simulink model "SMC"  (R2013b)
settings: Solver=ode45  StartTime=0.0  StopTime=50  RelTol=1e-3
InitFcn:
  | params
StartFcn:
  | params
undefined symbols (not defined in the file or in its folder): P, SM_controller
settings Model: Creator=dave  LastModifiedBy=dave
settings DataIOCC: SignalLoggingSaveFormat=ModelDataLogs  SignalLoggingName=sigsOut
settings DebuggingCC: SaveWithParameterizedLinksMsg=none  SignalResolutionControl=TryResolveAllWithWarning  SolverPrmCheckMsg=none  MultiTaskDSMMsg=warning  MultiTaskCondExecSysMsg=none
settings HardwareCC: TargetUnknown=on
settings RTWCC: IncludeERTFirstTime=on
settings GRTTargetCC: CombineOutputUpdateFcns=off  GRTInterface=on

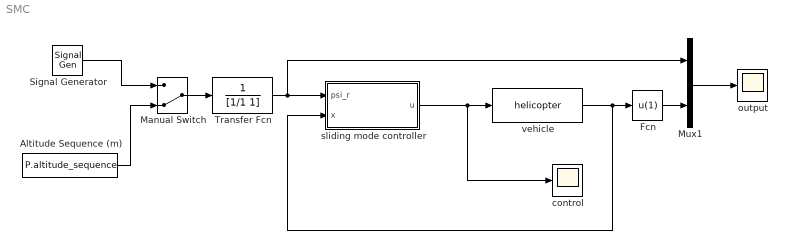
== system SMC ==
  Altitude Sequence (m) : FromWorkspace  VariableName=P.altitude_sequence  SampleTime=0
  Fcn : Fcn  Expr=u(1)
  Manual Switch : ManualSwitch  CurrentSetting=0
  Mux1 : Mux  Inputs=2
  Signal Generator : SignalGenerator  WaveForm=square  Amplitude=0.5  Frequency=.1
  Transfer Fcn : TransferFcn  Denominator=[1/1 1]
  control : Scope
      settings: YMin=-25  YMax=50
  output : Scope
      settings: YMin=0  YMax=0.8
  sliding mode controller : Subsystem
  vehicle : S-Function  FunctionName=helicopter  Parameters=P  EnableBusSupport=off
  wires:
  vehicle/1 -> sliding mode controller/2(x), Fcn/1
  Mux1/1 -> output/1
  sliding mode controller/1(u) -> vehicle/1, control/1
  Fcn/1 -> Mux1/2
  Transfer Fcn/1 -> Mux1/1, sliding mode controller/1(psi_r)
  Manual Switch/1 -> Transfer Fcn/1
  Signal Generator/1 -> Manual Switch/1
  Altitude Sequence (m)/1 -> Manual Switch/2

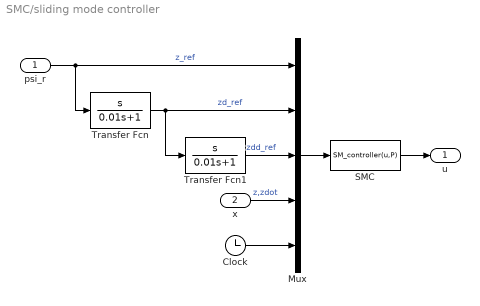
== system SMC/sliding mode controller ==
  psi_r : Inport
  x : Inport  Port=2
  Clock : Clock
  Mux : Mux  Inputs=5
  SMC : MATLABFcn  MATLABFcn=SM_controller(u,P)  SampleTime=P.Ts
  Transfer Fcn : TransferFcn  Numerator=[1 0]  Denominator=[0.01 1]
  Transfer Fcn1 : TransferFcn  Numerator=[1 0]  Denominator=[0.01 1]
  u : Outport
  wires:
  psi_r/1 -> Mux/1, Transfer Fcn/1  "z_ref"
  Transfer Fcn/1 -> Transfer Fcn1/1, Mux/2  "zd_ref"
  Transfer Fcn1/1 -> Mux/3  "zdd_ref"
  Mux/1 -> SMC/1
  x/1 -> Mux/4  "z,zdot"
  Clock/1 -> Mux/5
  SMC/1 -> u/1
